simulink model "MultipleAgentsChoice_NoVR"  (Simulink 7.5)
settings: Solver=ode45  StartTime=0.0  StopTime=1000  RelTol=1e-4  AbsTol=1e-4
libraries: simulink x64
(part 1 of 6)
Description:
  | % Copyright (C) 2012 Nicholas K. Lincoln, Sandor M. Veres, Louise Dennis,
  | % Michael Fisher, and Alexei Lisitsa.
  | %
  | % This file is part of the EASS (Engineering Autonomous Space Software)
  | % Demonstrator Set.
  | %
  | % The EASS Demonstrator Set is free software: you can redistribute it
  | % and/or modify it under the terms of the GNU Lesser General Public License
  | % as published by the Free Software Foundation, either version 3 of the
  | % License, or (at your option) any later version.
  | %
  | % The EASS Demonstrator Set is distributed in the hope that it will be
  | % useful, but WITHOUT ANY WARRANTY; without even the implied warranty of
  | % MERCHANTABILITY or FITNESS FOR A PARTICULAR PURPOSE.  See the GNU Lesser
  | % General Public License for more details.
  | %
  | % You should have received a copy of the GNU Lesser General Public License
  | % along with the EASS Demonstrator Set.  If not, see
  | % <http://www.gnu.org/licenses/>.
settings Model: Creator=N K Lincoln  LastModifiedBy=lad
settings SolverCC: ZeroCrossControl=DisableAll
settings OptimizationCC: InitFltsAndDblsToZero=on
settings DebuggingCC: ReadBeforeWriteMsg=DisableAll  WriteAfterWriteMsg=DisableAll  WriteAfterReadMsg=DisableAll  SaveWithParameterizedLinksMsg=none  SignalResolutionControl=TryResolveAllWithWarning  SolverPrmCheckMsg=none  InheritedTsInSrcMsg=none  StrictBusMsg=Warning
settings HardwareCC: TargetHWDeviceType=32-bit Generic
settings GRTTargetCC: TargetFcnLib=ansi_tfl_tmw.mat

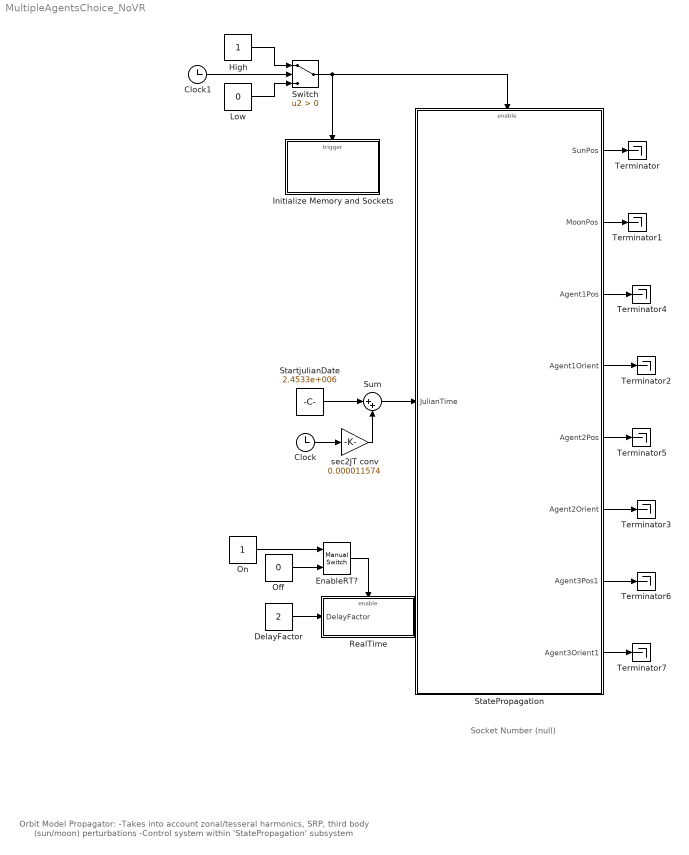
== system MultipleAgentsChoice_NoVR ==
  note: Orbit Model Propagator:
      | -Takes into account zonal/tesseral harmonics, SRP, third body (sun/moon) perturbations
      | -Control system within 'StatePropagation' subsystem
  note: Socket Number (null)
  Clock : Clock
      settings: Decimation=10
  Clock1 : Clock
      settings: Decimation=10
  DelayFactor : Constant  Value=2  OutDataType=sfix(16)  OutScaling=2^0
  EnableRT? : simulink/Signal Routing/Manual Switch  SystemSampleTime=-1  sw=1  action=0  varsize=off
  High : Constant  OutDataType=sfix(16)  OutScaling=2^0
  Initialize Memory and Sockets : Subsystem  TreatAsAtomicUnit=on
  Low : Constant  Value=0  OutDataType=sfix(16)  OutScaling=2^0
  Off : Constant  Value=0  OutDataType=sfix(16)  OutScaling=2^0
  On : Constant  OutDataType=sfix(16)  OutScaling=2^0
  RealTime : Subsystem
  StartjulianDate : Constant  Value=2.4533e+006  OutDataType=sfix(16)  OutScaling=2^0
  StatePropagation : Subsystem
  Sum : Sum  Inputs=|++  OutDataType=sfix(16)  OutScaling=2^0
  Switch : Switch  Criteria=u2 > Threshold
  Terminator{,1..7} (8 alike) : Terminator
  sec2JT conv : Gain  Gain=0.000011574  ParameterDataType=sfix(16)  ParameterScaling=2^0  OutDataType=sfix(16)  OutScaling=2^0
  wires:
  Clock/1 -> sec2JT conv/1
  sec2JT conv/1 -> Sum/2
  Sum/1 -> StatePropagation/1(JulianTime)
  StartjulianDate/1 -> Sum/1
  StatePropagation/7(Agent3Pos1) -> Terminator6/1
  StatePropagation/8(Agent3Orient1) -> Terminator7/1
  StatePropagation/6(Agent2Orient) -> Terminator3/1
  StatePropagation/5(Agent2Pos) -> Terminator5/1
  StatePropagation/4(Agent1Orient) -> Terminator2/1
  StatePropagation/3(Agent1Pos) -> Terminator4/1
  StatePropagation/1(SunPos) -> Terminator/1
  StatePropagation/2(MoonPos) -> Terminator1/1
  On/1 -> EnableRT?/1
  Off/1 -> EnableRT?/2
  EnableRT?/1 -> RealTime/Enable
  DelayFactor/1 -> RealTime/1(DelayFactor)
  Low/1 -> Switch/3
  High/1 -> Switch/1
  Clock1/1 -> Switch/2
  Switch/1 -> StatePropagation/Enable, Initialize Memory and Sockets/Trigger

== system MultipleAgentsChoice_NoVR/Initialize Memory and Sockets ==
  note: number of agents in the cluster
  Trigger : TriggerPort
  Constant : Constant  Value=3  OutDataType=fixdt(1, 16)  OutScaling=2^0
  create multi memory : MATLABFcn  MATLABFcn=create_agent_memory_multi  OutputDimensions=0
  wires:
  Constant/1 -> create multi memory/1

== system MultipleAgentsChoice_NoVR/RealTime ==
  DelayFactor : Inport  OutDataType=sfix(16)  OutScaling=2^0
  Enable : EnablePort
  Real-time synchronization : Subsystem
  wires:
  DelayFactor/1 -> Real-time synchronization/1(DelayFactor)

== system MultipleAgentsChoice_NoVR/StatePropagation ==
  JulianTime : Inport  OutDataType=sfix(16)  OutScaling=2^0
  Enable : EnablePort
  BodyAccelerations : Subsystem
  Bus Selector : BusSelector  OutputSignals=SunPos,MoonPos
  Bus Selector1 : BusSelector  OutputSignals=Agent1Pos,Agent1Vel,Agent2Pos,Agent2Vel,Agent3Pos,Agent3Vel
  MATLAB Fcn : MATLABFcn  MATLABFcn=SatOrient  OutputDimensions=4
  MATLAB Fcn2 : MATLABFcn  MATLABFcn=SatOrient  OutputDimensions=4
  MATLAB Fcn3 : MATLABFcn  MATLABFcn=SatOrient  OutputDimensions=4
  Mux : Mux  Inputs=2
  Mux2 : Mux  Inputs=2
  Mux3 : Mux  Inputs=2
  PropogateAgents : Subsystem
  SatelliteControlAccel : Subsystem
  SunPos : Outport  OutDataType=sfix(16)  OutScaling=2^0
  MoonPos : Outport  Port=2  OutDataType=sfix(16)  OutScaling=2^0
  Agent1Pos : Outport  Port=3  OutDataType=sfix(16)  OutScaling=2^0
  Agent1Orient : Outport  Port=4  OutDataType=sfix(16)  OutScaling=2^0
  Agent2Pos : Outport  Port=5  OutDataType=sfix(16)  OutScaling=2^0
  Agent2Orient : Outport  Port=6  OutDataType=sfix(16)  OutScaling=2^0
  Agent3Pos1 : Outport  Port=7  OutDataType=sfix(16)  OutScaling=2^0
  Agent3Orient1 : Outport  Port=8  OutDataType=sfix(16)  OutScaling=2^0
  wires:
  SatelliteControlAccel/1(AccelControl) -> PropogateAgents/2(ControlAccelrations)
  JulianTime/1 -> BodyAccelerations/1(JulianTime)
  BodyAccelerations/2(SunMoonPos) -> [SunMoonPos]
  BodyAccelerations/1(BodyAccelerations) -> PropogateAgents/1(BodyAccelerations)
  [SunMoonPos] -> Bus Selector/1
  Bus Selector/1 -> SunPos/1  "<SunPos>"
  Bus Selector/2 -> MoonPos/1  "<MoonPos>"
  PropogateAgents/1(GEOC_current) -> Bus Selector1/1, BodyAccelerations/2(GEOC_Current), SatelliteControlAccel/1(GEOC_Current)
  Bus Selector1/1 -> Agent1Pos/1, Mux/1  "<Agent1Pos>"
  Bus Selector1/3 -> Agent2Pos/1, Mux2/1  "<Agent2Pos>"
  Bus Selector1/2 -> Mux/2  "<Agent1Vel>"
  Bus Selector1/4 -> Mux2/2  "<Agent2Vel>"
  Mux/1 -> MATLAB Fcn/1
  Mux2/1 -> MATLAB Fcn2/1
  MATLAB Fcn/1 -> Agent1Orient/1
  MATLAB Fcn2/1 -> Agent2Orient/1
  Bus Selector1/5 -> Mux3/1, Agent3Pos1/1  "<Agent3Pos>"
  Bus Selector1/6 -> Mux3/2  "<Agent3Vel>"
  Mux3/1 -> MATLAB Fcn3/1
  MATLAB Fcn3/1 -> Agent3Orient1/1
  SatelliteControlAccel/2(InitialConditions) -> PropogateAgents/3(InitialConditions)

== system MultipleAgentsChoice_NoVR/RealTime/Real-time synchronization ==
  DelayFactor : Inport  OutDataType=sfix(16)  OutScaling=2^0
  Clock : Clock
      settings: Decimation=10
  Real-time Synchronization : Subsystem
  wires:
  Clock/1 -> Real-time Synchronization/1(run)
  DelayFactor/1 -> Real-time Synchronization/2(DelayFactor)

== system MultipleAgentsChoice_NoVR/StatePropagation/BodyAccelerations ==
  note: THIS IS THE DYNAMIC REGIME INFLUENCING AGENT MOTION
  JulianTime : Inport  OutDataType=sfix(16)  OutScaling=2^0
  GEOC_Current : Inport  Port=2  OutDataType=sfix(16)  OutScaling=2^0
  Agent1 : Subsystem
  Agent2 : Subsystem
  Agent3 : Subsystem
  Bus Creator : BusCreator  Inputs=3
  Bus Creator1 : BusCreator  Inputs=2
  Bus Selector : BusSelector  OutputSignals=Agent1Pos,Agent2Pos,Agent3Pos
  MoonPos : Subsystem
  SunPos : Subsystem
  BodyAccelerations : Outport  OutDataType=sfix(16)  OutScaling=2^0
  SunMoonPos : Outport  Port=2  OutDataType=sfix(16)  OutScaling=2^0
  wires:
  JulianTime/1 -> MoonPos/1(JT), SunPos/1(JT), Agent1/1(JT), Agent2/1(JT), Agent3/1(JT)
  Agent1/1(A1Accels) -> Bus Creator/1  "Agent1"
  Agent2/1(A2Accels) -> Bus Creator/2  "Agent2"
  Bus Creator/1 -> BodyAccelerations/1
  MoonPos/1(MoonGEOC_Pos) -> Bus Creator1/1  "MoonPos"
  SunPos/1(SunPos) -> Bus Creator1/2  "SunPos"
  Bus Creator1/1 -> SunMoonPos/1
  GEOC_Current/1 -> Bus Selector/1
  Bus Selector/1 -> Agent1/2(A1GEOC_Pos)  "<Agent1Pos>"
  Bus Selector/2 -> Agent2/2(A2GEOC_Pos)  "<Agent2Pos>"
  Agent3/1(A3Accels) -> Bus Creator/3  "Agent3"
  Bus Selector/3 -> Agent3/2(A3GEOC_Pos)  "<Agent3Pos>"

== system MultipleAgentsChoice_NoVR/StatePropagation/PropogateAgents ==
  BodyAccelerations : Inport  OutDataType=sfix(16)  OutScaling=2^0
  ControlAccelrations : Inport  Port=2  OutDataType=sfix(16)  OutScaling=2^0
  InitialConditions : Inport  Port=3  OutDataType=sfix(16)  OutScaling=2^0
  Agent1 : Subsystem
  Agent2 : Subsystem
  Agent3 : Subsystem
  Bus Creator : BusCreator  Inputs=6
  Bus Selector : BusSelector  OutputSignals=Agent1,Agent2,Agent3
  Bus Selector1 : BusSelector  OutputSignals=Agent1,Agent2,Agent3
  Bus Selector2 : BusSelector  OutputSignals=ECI_A1,ECI_A2,ECI_A3
  Sum : Sum  Inputs=|++  OutDataType=sfix(16)  OutScaling=2^0
  Sum1 : Sum  Inputs=|++  OutDataType=sfix(16)  OutScaling=2^0
  Sum2 : Sum  Inputs=|++  OutDataType=sfix(16)  OutScaling=2^0
  GEOC_current : Outport  OutDataType=sfix(16)  OutScaling=2^0
  wires:
  BodyAccelerations/1 -> Bus Selector/1
  InitialConditions/1 -> Bus Selector1/1
  Bus Creator/1 -> GEOC_current/1  "GEOC_Current"
  Agent1/1(GEOC_Pos) -> Bus Creator/1  "Agent1Pos"
  Agent2/1(GEOC_Pos) -> Bus Creator/3  "Agent2Pos"
  Agent1/2(GEOC_Vel) -> Bus Creator/2  "Agent1Vel"
  Agent2/2(GEOC_Vel) -> Bus Creator/4  "Agent2Vel"
  ControlAccelrations/1 -> Bus Selector2/1
  Sum/1 -> Agent1/1(Accelerations)
  Sum1/1 -> Agent2/1(Accelerations)
  Bus Selector/1 -> Sum/1  "<Agent1>"
  Bus Selector/2 -> Sum1/1  "<Agent2>"
  Bus Selector2/1 -> Sum/2  "<ECI_A1>"
  Bus Selector2/2 -> Sum1/2  "<ECI_A2>"
  Bus Selector1/2 -> Agent2/2(InitialConditions)  "<Agent2>"
  Bus Selector1/1 -> Agent1/2(InitialConditions)  "<Agent1>"
  Agent3/1(GEOC_Pos) -> Bus Creator/5  "Agent3Pos"
  Agent3/2(GEOC_Vel) -> Bus Creator/6  "Agent3Vel"
  Sum2/1 -> Agent3/1(Accelerations)
  Bus Selector2/3 -> Sum2/2  "<ECI_A3>"
  Bus Selector/3 -> Sum2/1  "<Agent3>"
  Bus Selector1/3 -> Agent3/2(InitialConditions)  "<Agent3>"

== system MultipleAgentsChoice_NoVR/StatePropagation/SatelliteControlAccel ==
  GEOC_Current : Inport  OutDataType=sfix(16)  OutScaling=2^0
  Agent Body1 : Subsystem
  Agent Body2 : Subsystem
  Agent Body3 : Subsystem
  Agent1 : Constant  OutDataType=sfix(16)  OutScaling=2^0
  Agent2 : Constant  Value=2  OutDataType=sfix(16)  OutScaling=2^0
  Agent3 : Constant  Value=3  OutDataType=sfix(16)  OutScaling=2^0
  BodyToOrbitFrameConvert : Subsystem
  Bus Creator : BusCreator  Inputs=3
  Bus Creator1 : BusCreator  Inputs=3
  Bus Selector : BusSelector  OutputSignals=A1Commands,A2Commands,A3Commands,LeadAgent
  Data Type Conversion : DataTypeConversion  OutDataType=sfix(16)  OutScaling=2^0
  Data Type Conversion1 : DataTypeConversion  OutDataType=sfix(16)  OutScaling=2^0
  GetCmdAIL : Subsystem
  InitialErrors : Subsystem
  NoSend : Constant  Value=0  OutDataType=sfix(16)  OutScaling=2^0
  NoSend1 : Constant  Value=0  OutDataType=sfix(16)  OutScaling=2^0
  Pulse Generator : DiscretePulseGenerator  PulseType=Time based  Amplitude=1  Period=1  PulseWidth=50  PhaseDelay=0  SampleTime=1
  Pulse Generator1 : DiscretePulseGenerator  PulseType=Time based  Amplitude=1  Period=0.1  PulseWidth=50  PhaseDelay=0  SampleTime=1
  Selective Hill State Provision and Discretisation : Subsystem
  TriggeredSendAgent : Subsystem  TreatAsAtomicUnit=on
  TriggeredSendCont : Subsystem  TreatAsAtomicUnit=on
  TurnOff : simulink/Signal Routing/Manual Switch  SystemSampleTime=-1  sw=1  action=0  varsize=off
  TurnOff1 : simulink/Signal Routing/Manual Switch  SystemSampleTime=-1  sw=1  action=0  varsize=off
  AccelControl : Outport  OutDataType=sfix(16)  OutScaling=2^0
  InitialConditions : Outport  Port=2  OutDataType=sfix(16)  OutScaling=2^0
  wires:
  BodyToOrbitFrameConvert/1(GlobalAccel) -> AccelControl/1
  GEOC_Current/1 -> Selective Hill State Provision and Discretisation/1(GEOC_Current), BodyToOrbitFrameConvert/3(GEOC_Current)
  Selective Hill State Provision and Discretisation/1(HillState) -> Agent Body1/2(StateInformation), Agent Body2/2(StateInformation), Agent Body3/2(StateInformation)
  Agent Body1/1(AccelA1) -> Bus Creator/1
  Bus Creator/1 -> BodyToOrbitFrameConvert/1(BodyAccel)
  Bus Selector/1 -> Agent Body1/1(Commands)  "<A1Commands>"
  Bus Selector/2 -> Agent Body2/1(Commands)  "<A2Commands>"
  Agent Body2/1(AccelA2) -> Bus Creator/2
  Agent Body1/2(A1Data) -> Bus Creator1/1
  Agent Body2/2(A2Data) -> Bus Creator1/2
  Bus Creator1/1 -> TriggeredSendAgent/1(Data), TriggeredSendCont/1(Data)
  Data Type Conversion/1 -> TriggeredSendAgent/Trigger
  NoSend/1 -> TurnOff/2
  TurnOff/1 -> Data Type Conversion/1
  Pulse Generator/1 -> TurnOff/1
  GetCmdAIL/1(Commands2) -> Bus Selector/1
  Bus Selector/3 -> Agent Body3/1(Commands)  "<A3Commands>"
  Agent Body3/1(AccelA3) -> Bus Creator/3
  Agent Body3/2(A3Data) -> Bus Creator1/3
  Bus Selector/4 -> Selective Hill State Provision and Discretisation/2(LeadAgent), BodyToOrbitFrameConvert/2(LeadAgent)  "<LeadAgent>"
  InitialErrors/1(Out1) -> InitialConditions/1
  Agent2/1 -> Agent Body2/3(AgentNumber)
  Agent3/1 -> Agent Body3/3(AgentNumber)
  Agent1/1 -> Agent Body1/3(AgentNumber)
  NoSend1/1 -> TurnOff1/2
  TurnOff1/1 -> Data Type Conversion1/1
  Pulse Generator1/1 -> TurnOff1/1
  Data Type Conversion1/1 -> TriggeredSendCont/Trigger

== system MultipleAgentsChoice_NoVR/RealTime/Real-time synchronization/Real-time Synchronization ==
  run : Inport
  DelayFactor : Inport  Port=2  OutDataType=sfix(16)  OutScaling=2^0
  Clock : Clock
      settings: Decimation=10
  Product : Product  OutDataType=sfix(16)  OutScaling=2^0  RndMeth=Zero
  Subsystem : Subsystem  TreatAsAtomicUnit=on
  Sum : Sum  Inputs=+-  SaturateOnIntegerOverflow=on  InputSameDT=on  OutDataTypeStr=Inherit: Same as first input
  real-time synchronization : MATLABFcn  MATLABFcn=waitfortreal  OutputDimensions=0
  wires:
  run/1 -> Subsystem/Trigger
  Subsystem/1(Out) -> Sum/2
  Clock/1 -> Sum/1, Subsystem/1(In)
  Sum/1 -> Product/2
  Product/1 -> real-time synchronization/1
  DelayFactor/1 -> Product/1

== system MultipleAgentsChoice_NoVR/StatePropagation/BodyAccelerations/Agent1 ==
  JT : Inport  OutDataType=sfix(16)  OutScaling=2^0
  A1GEOC_Pos : Inport  Port=2  OutDataType=sfix(16)  OutScaling=2^0
  EarthAccel(J2) : Subsystem
  EarthAccel1 : Subsystem
  Gain{,1..3,5} (5 alike) : Gain  ParameterDataType=sfix(16)  ParameterScaling=2^0  OutDataType=sfix(16)  OutScaling=2^0
  Manual Switch : simulink/Signal Routing/Manual Switch  SystemSampleTime=-1  sw=1  action=0  varsize=off
  MoonAccel : Subsystem
  SRPAccel : Subsystem
  Sum : Sum  Inputs=|++++  OutDataType=sfix(16)  OutScaling=2^0
  SunAccel : Subsystem
  A1Accels : Outport  OutDataType=sfix(16)  OutScaling=2^0
  wires:
  EarthAccel(J2)/1(AccelEarth) -> Gain/1
  MoonAccel/1(AccelMoon) -> Gain1/1
  SRPAccel/1(AccelSRP) -> Gain2/1
  SunAccel/1(AccelSun) -> Gain5/1
  EarthAccel1/1(AccelEarth) -> Gain3/1
  A1GEOC_Pos/1 -> EarthAccel1/1(GEOC_Pos), EarthAccel(J2)/2(GEOC_Pos), MoonAccel/2(SatGEOC_Pos), SRPAccel/2(GEOC_Pos1), SunAccel/2(SatGEOC_Pos1)
  JT/1 -> EarthAccel(J2)/1(JT), MoonAccel/1(JT), SRPAccel/1(JT1), SunAccel/1(JT1)
  Gain/1 -> Sum/1
  Gain1/1 -> Sum/2
  Gain2/1 -> Sum/3
  Gain5/1 -> Sum/4
  Sum/1 -> Manual Switch/2
  Manual Switch/1 -> A1Accels/1
  Gain3/1 -> Manual Switch/1

== system MultipleAgentsChoice_NoVR/StatePropagation/BodyAccelerations/Agent2 ==
  JT : Inport  OutDataType=sfix(16)  OutScaling=2^0
  A2GEOC_Pos : Inport  Port=2  OutDataType=sfix(16)  OutScaling=2^0
  EarthAccel(J2) : Subsystem
  EarthAccel1 : Subsystem
  Gain{,1..3,5} (5 alike) : Gain  ParameterDataType=sfix(16)  ParameterScaling=2^0  OutDataType=sfix(16)  OutScaling=2^0
  Manual Switch : simulink/Signal Routing/Manual Switch  SystemSampleTime=-1  sw=1  action=0  varsize=off
  MoonAccel : Subsystem
  SRPAccel : Subsystem
  Sum : Sum  Inputs=|++++  OutDataType=sfix(16)  OutScaling=2^0
  SunAccel : Subsystem
  A2Accels : Outport  OutDataType=sfix(16)  OutScaling=2^0
  wires:
  Gain3/1 -> Manual Switch/1
  Manual Switch/1 -> A2Accels/1
  Sum/1 -> Manual Switch/2
  Gain5/1 -> Sum/4
  Gain2/1 -> Sum/3
  Gain1/1 -> Sum/2
  Gain/1 -> Sum/1
  JT/1 -> SunAccel/1(JT1), SRPAccel/1(JT1), MoonAccel/1(JT), EarthAccel(J2)/1(JT)
  A2GEOC_Pos/1 -> SunAccel/2(SatGEOC_Pos1), SRPAccel/2(GEOC_Pos1), MoonAccel/2(SatGEOC_Pos), EarthAccel(J2)/2(GEOC_Pos), EarthAccel1/1(GEOC_Pos)
  EarthAccel1/1(AccelEarth) -> Gain3/1
  SunAccel/1(AccelSun) -> Gain5/1
  SRPAccel/1(AccelSRP) -> Gain2/1
  MoonAccel/1(AccelMoon) -> Gain1/1
  EarthAccel(J2)/1(AccelEarth) -> Gain/1

== system MultipleAgentsChoice_NoVR/StatePropagation/BodyAccelerations/Agent3 ==
  JT : Inport  OutDataType=sfix(16)  OutScaling=2^0
  A3GEOC_Pos : Inport  Port=2  OutDataType=sfix(16)  OutScaling=2^0
  EarthAccel(J2) : Subsystem
  EarthAccel1 : Subsystem
  Gain{,1..3,5} (5 alike) : Gain  ParameterDataType=sfix(16)  ParameterScaling=2^0  OutDataType=sfix(16)  OutScaling=2^0
  Manual Switch : simulink/Signal Routing/Manual Switch  SystemSampleTime=-1  sw=1  action=0  varsize=off
  MoonAccel : Subsystem
  SRPAccel : Subsystem
  Sum : Sum  Inputs=|++++  OutDataType=sfix(16)  OutScaling=2^0
  SunAccel : Subsystem
  A3Accels : Outport  OutDataType=sfix(16)  OutScaling=2^0
  wires:
  EarthAccel(J2)/1(AccelEarth) -> Gain/1
  MoonAccel/1(AccelMoon) -> Gain1/1
  SRPAccel/1(AccelSRP) -> Gain2/1
  SunAccel/1(AccelSun) -> Gain5/1
  EarthAccel1/1(AccelEarth) -> Gain3/1
  A3GEOC_Pos/1 -> EarthAccel1/1(GEOC_Pos), EarthAccel(J2)/2(GEOC_Pos), MoonAccel/2(SatGEOC_Pos), SRPAccel/2(GEOC_Pos1), SunAccel/2(SatGEOC_Pos1)
  JT/1 -> EarthAccel(J2)/1(JT), MoonAccel/1(JT), SRPAccel/1(JT1), SunAccel/1(JT1)
  Gain/1 -> Sum/1
  Gain1/1 -> Sum/2
  Gain2/1 -> Sum/3
  Gain5/1 -> Sum/4
  Sum/1 -> Manual Switch/2
  Manual Switch/1 -> A3Accels/1
  Gain3/1 -> Manual Switch/1

== system MultipleAgentsChoice_NoVR/StatePropagation/BodyAccelerations/MoonPos ==
  JT : Inport  OutDataType=sfix(16)  OutScaling=2^0
  MoonDirVector : MATLABFcn  MATLABFcn=moon
  Re : Gain  Gain=6371  ParameterDataType=sfix(16)  ParameterScaling=2^0  OutDataType=sfix(16)  OutScaling=2^0
  MoonGEOC_Pos : Outport  OutDataType=sfix(16)  OutScaling=2^0
  wires:
  Re/1 -> MoonGEOC_Pos/1
  MoonDirVector/1 -> Re/1
  JT/1 -> MoonDirVector/1

== system MultipleAgentsChoice_NoVR/StatePropagation/BodyAccelerations/SunPos ==
  JT : Inport  OutDataType=sfix(16)  OutScaling=2^0
  AU : Gain  Gain=1.4960e8  ParameterDataType=sfix(16)  ParameterScaling=2^0  OutDataType=sfix(16)  OutScaling=2^0
  SunDirVector : MATLABFcn  MATLABFcn=sun
  SunPos : Outport  OutDataType=sfix(16)  OutScaling=2^0
  wires:
  AU/1 -> SunPos/1
  SunDirVector/1 -> AU/1
  JT/1 -> SunDirVector/1

== system MultipleAgentsChoice_NoVR/StatePropagation/PropogateAgents/Agent1 ==
  Accelerations : Inport  OutDataType=sfix(16)  OutScaling=2^0
  InitialConditions : Inport  Port=2  OutDataType=sfix(16)  OutScaling=2^0
  Demux : Demux  Outputs=6
  Integrate2Pos : Integrator  InitialConditionSource=external
  Integrate2Vel : Integrator  InitialConditionSource=external
  Mux : Mux  Inputs=3
  Mux1 : Mux  Inputs=3
  GEOC_Pos : Outport  OutDataType=sfix(16)  OutScaling=2^0
  GEOC_Vel : Outport  Port=2  OutDataType=sfix(16)  OutScaling=2^0
  wires:
  Integrate2Vel/1 -> Integrate2Pos/1, GEOC_Vel/1
  Accelerations/1 -> Integrate2Vel/1
  Demux/1 -> Mux/1
  Demux/2 -> Mux/2
  Demux/3 -> Mux/3
  Demux/4 -> Mux1/1
  Demux/5 -> Mux1/2
  Demux/6 -> Mux1/3
  InitialConditions/1 -> Demux/1
  Mux1/1 -> Integrate2Vel/2
  Mux/1 -> Integrate2Pos/2
  Integrate2Pos/1 -> GEOC_Pos/1

== system MultipleAgentsChoice_NoVR/StatePropagation/PropogateAgents/Agent2 ==
  Accelerations : Inport  OutDataType=sfix(16)  OutScaling=2^0
  InitialConditions : Inport  Port=2  OutDataType=sfix(16)  OutScaling=2^0
  Demux : Demux  Outputs=6
  Integrate2Pos : Integrator  InitialConditionSource=external
  Integrate2Vel : Integrator  InitialConditionSource=external
  Mux : Mux  Inputs=3
  Mux1 : Mux  Inputs=3
  GEOC_Pos : Outport  OutDataType=sfix(16)  OutScaling=2^0
  GEOC_Vel : Outport  Port=2  OutDataType=sfix(16)  OutScaling=2^0
  wires:
  Integrate2Pos/1 -> GEOC_Pos/1
  Mux/1 -> Integrate2Pos/2
  Mux1/1 -> Integrate2Vel/2
  InitialConditions/1 -> Demux/1
  Demux/6 -> Mux1/3
  Demux/5 -> Mux1/2
  Demux/4 -> Mux1/1
  Demux/3 -> Mux/3
  Demux/2 -> Mux/2
  Demux/1 -> Mux/1
  Accelerations/1 -> Integrate2Vel/1
  Integrate2Vel/1 -> GEOC_Vel/1, Integrate2Pos/1

== system MultipleAgentsChoice_NoVR/StatePropagation/PropogateAgents/Agent3 ==
  Accelerations : Inport  OutDataType=sfix(16)  OutScaling=2^0
  InitialConditions : Inport  Port=2  OutDataType=sfix(16)  OutScaling=2^0
  Demux : Demux  Outputs=6
  Integrate2Pos : Integrator  InitialConditionSource=external
  Integrate2Vel : Integrator  InitialConditionSource=external
  Mux : Mux  Inputs=3
  Mux1 : Mux  Inputs=3
  GEOC_Pos : Outport  OutDataType=sfix(16)  OutScaling=2^0
  GEOC_Vel : Outport  Port=2  OutDataType=sfix(16)  OutScaling=2^0
  wires:
  Integrate2Vel/1 -> Integrate2Pos/1, GEOC_Vel/1
  Accelerations/1 -> Integrate2Vel/1
  Demux/1 -> Mux/1
  Demux/2 -> Mux/2
  Demux/3 -> Mux/3
  Demux/4 -> Mux1/1
  Demux/5 -> Mux1/2
  Demux/6 -> Mux1/3
  InitialConditions/1 -> Demux/1
  Mux1/1 -> Integrate2Vel/2
  Mux/1 -> Integrate2Pos/2
  Integrate2Pos/1 -> GEOC_Pos/1

== system MultipleAgentsChoice_NoVR/StatePropagation/SatelliteControlAccel/Agent Body1 ==
  note: 1=sequence running
  note: 0=no sequence ruinning
  Commands : Inport  OutDataType=sfix(16)  OutScaling=2^0
  StateInformation : Inport  Port=2  OutDataType=sfix(16)  OutScaling=2^0
  AgentNumber : Inport  Port=3  OutDataType=sfix(16)  OutScaling=2^0
  Actual Thruster response : Subsystem
  ActualForces : Display
  AgentNumber1 : InportShadow  Port=3  OutDataType=sfix(16)  OutScaling=2^0
  Bus Creator : BusCreator  Inputs=9
  Bus Creator1 : BusCreator  Inputs=2
  Bus Creator2 : BusCreator  Inputs=9
  Bus Selector : BusSelector  OutputSignals=ControlType,UseX,UseY,UseZ,UseXYZ,XValves1,XSwitch1,YValves,YSwitch,ZValves,ZSwitch,XYZValves,XYZSwitch,A1Break
  Bus Selector1 : BusSelector  OutputSignals=A1HillState.HillPosCont,A1HillState.HillVelCont,A1HillState.HillPosDisc,A1HillState.HillVelDisc
  Clock : Clock
      settings: Decimation=10
  Constant : Constant  Value=[0;0;0]  OutDataType=sfix(16)  OutScaling=2^0
  Convert2Accels : Subsystem
  Demux : Demux  Outputs=8
  Derivative : Derivative
  DesiredForces : Display
  Mux : Mux  Inputs=6
  Mux1 : Mux
  Mux2 : Mux
  Mux3 : Mux  Inputs=3
  Mux4 : Mux  Inputs=2
  Mux5 : Mux  Inputs=2
  Plan : Display
  Sum : Sum  Inputs=|++  OutDataType=sfix(16)  OutScaling=2^0
  obtain_forcesXYZ_multi : MATLABFcn  MATLABFcn=obtain_forcesXYZ_multi  OutputDimensions=8
  AccelA1 : Outport  OutDataType=sfix(16)  OutScaling=2^0
  A1Data : Outport  Port=2  OutDataType=sfix(16)  OutScaling=2^0
  wires:
  Derivative/1 -> Mux/3
  Clock/1 -> Mux/4
  [CTstate] -> Derivative/1, Mux/2
  obtain_forcesXYZ_multi/1 -> Demux/1
  Mux/1 -> obtain_forcesXYZ_multi/1
  Bus Creator1/1 -> Actual Thruster response/1(Signals)
  Commands/1 -> Bus Selector/1
  Actual Thruster response/5(Forces) -> Bus Creator2/7, Sum/1, ActualForces/1  "A1ActualForces"
  Mux1/1 -> Bus Creator1/1  "A1ControlSignals"
  StateInformation/1 -> Bus Selector1/1
  Bus Selector1/1 -> Mux4/1  "<HillPosCont>"
  Bus Selector1/2 -> Mux4/2  "<HillVelCont>"
  Bus Selector1/3 -> Mux5/1  "<HillPosDisc>"
  Bus Selector1/4 -> Mux5/2  "<HillVelDisc>"
  Mux5/1 -> [DTstate]
  Mux4/1 -> [CTstate]
  Convert2Accels/1(Accels) -> AccelA1/1  "A1Accels"
  Actual Thruster response/2(YThrusterData) -> Bus Creator2/4  "A1YthrusterData"
  Actual Thruster response/1(XThrusterData) -> Bus Creator2/3  "A1XthrusterData"
  Actual Thruster response/3(ZThrusterData) -> Bus Creator2/5  "A1ZthrusterData"
  Demux/1 -> Bus Creator2/1, Plan/1  "A1PlanMsg"
  Bus Creator2/1 -> A1Data/1  "A1Data"
  [DTstate] -> Bus Creator2/9  "A1DTstate"
  Actual Thruster response/4(XYZThrusterData) -> Bus Creator2/6  "A1XYZthrusterData"
  Bus Selector/1 -> Mux/1  "<ControlType>"
  Bus Selector/2 -> Mux2/1  "<UseX>"
  Bus Selector/3 -> Mux2/2  "<UseY>"
  Bus Selector/4 -> Mux2/3  "<UseZ>"
  Bus Selector/5 -> Mux2/4  "<UseXYZ>"
  Mux2/1 -> Mux/5
  Bus Creator/1 -> Bus Creator1/2  "ConfigurationSignals"
  Bus Selector/6 -> Bus Creator/1  "<XValves1>"
  Bus Selector/7 -> Bus Creator/2  "<XSwitch1>"
  Bus Selector/8 -> Bus Creator/3  "<YValves>"
  Bus Selector/9 -> Bus Creator/4  "<YSwitch>"
  Bus Selector/10 -> Bus Creator/5  "<ZValves>"
  Bus Selector/11 -> Bus Creator/6  "<ZSwitch>"
  Bus Selector/12 -> Bus Creator/7  "<XYZValves>"
  Bus Selector/13 -> Bus Creator/8  "<XYZSwitch>"
  Demux/2 -> Mux3/1
  Demux/3 -> Mux3/2
  Demux/4 -> Mux3/3
  Demux/5 -> Mux1/1
  Demux/6 -> Mux1/2
  Demux/7 -> Mux1/3
  Demux/8 -> Mux1/4
  Mux3/1 -> Bus Creator2/2, DesiredForces/1  "A1DesiredForces"
  Sum/1 -> Convert2Accels/1(Forces)
  Constant/1 -> Sum/2
  AgentNumber/1 -> Mux/6
  AgentNumber1/1 -> Actual Thruster response/2(AgentNumber)
  Actual Thruster response/6(PressureData) -> Bus Creator2/8  "A1PressureData"
  Bus Selector/14 -> Bus Creator/9  "<A1Break>"

== system MultipleAgentsChoice_NoVR/StatePropagation/SatelliteControlAccel/Agent Body2 ==
  Commands : Inport  OutDataType=sfix(16)  OutScaling=2^0
  StateInformation : Inport  Port=2  OutDataType=sfix(16)  OutScaling=2^0
  AgentNumber : Inport  Port=3  OutDataType=sfix(16)  OutScaling=2^0
  Actual Thruster response : Subsystem
  AgentNumber1 : InportShadow  Port=3  OutDataType=sfix(16)  OutScaling=2^0
  Bus Creator : BusCreator  Inputs=9
  Bus Creator1 : BusCreator  Inputs=2
  Bus Creator2 : BusCreator  Inputs=9
  Bus Selector : BusSelector  OutputSignals=ControlType,UseX,UseY,UseZ,UseXYZ,XValves1,XSwitch1,YValves,YSwitch,ZValves,ZSwitch,XYZValves,XYZSwitch,A2Break
  Bus Selector1 : BusSelector  OutputSignals=A2HillState.HillPosCont,A2HillState.HillVelCont,A2HillState.HillPosDisc,A2HillState.HillVelDisc
  Clock : Clock
      settings: Decimation=10
  Convert2Accels : Subsystem
  Demux : Demux  Outputs=8
  Derivative : Derivative
  Mux : Mux  Inputs=6
  Mux1 : Mux
  Mux2 : Mux
  Mux3 : Mux  Inputs=3
  Mux4 : Mux  Inputs=2
  Mux5 : Mux  Inputs=2
  obtain_forcesXYZ_multi : MATLABFcn  MATLABFcn=obtain_forcesXYZ_multi  OutputDimensions=8
  AccelA2 : Outport  OutDataType=sfix(16)  OutScaling=2^0
  A2Data : Outport  Port=2  OutDataType=sfix(16)  OutScaling=2^0
  wires:
  Bus Selector/13 -> Bus Creator/8  "<XYZSwitch>"
  Bus Selector/12 -> Bus Creator/7  "<XYZValves>"
  Bus Selector/11 -> Bus Creator/6  "<ZSwitch>"
  Bus Selector/10 -> Bus Creator/5  "<ZValves>"
  Bus Selector/9 -> Bus Creator/4  "<YSwitch>"
  Bus Selector/8 -> Bus Creator/3  "<YValves>"
  Bus Selector/7 -> Bus Creator/2  "<XSwitch1>"
  Bus Selector/6 -> Bus Creator/1  "<XValves1>"
  Bus Creator/1 -> Bus Creator1/2  "ConfigurationSignals"
  Mux2/1 -> Mux/5
  Bus Selector/5 -> Mux2/4  "<UseXYZ>"
  Bus Selector/4 -> Mux2/3  "<UseZ>"
  Bus Selector/3 -> Mux2/2  "<UseY>"
  Bus Selector/2 -> Mux2/1  "<UseX>"
  Bus Selector/1 -> Mux/1  "<ControlType>"
  Actual Thruster response/4(XYZThrusterData) -> Bus Creator2/6  "A2XYZthrusterData"
  [DTstate] -> Bus Creator2/9  "A2DTstate"
  Bus Creator2/1 -> A2Data/1  "A2Data"
  Actual Thruster response/3(ZThrusterData) -> Bus Creator2/5  "A2ZthrusterData"
  Actual Thruster response/1(XThrusterData) -> Bus Creator2/3  "A2XthrusterData"
  Actual Thruster response/2(YThrusterData) -> Bus Creator2/4  "A2YthrusterData"
  Convert2Accels/1(Accels) -> AccelA2/1  "A2Accels"
  Mux4/1 -> [CTstate]
  Mux5/1 -> [DTstate]
  Bus Selector1/4 -> Mux5/2  "<HillVelDisc>"
  Bus Selector1/3 -> Mux5/1  "<HillPosDisc>"
  Bus Selector1/2 -> Mux4/2  "<HillVelCont>"
  Bus Selector1/1 -> Mux4/1  "<HillPosCont>"
  StateInformation/1 -> Bus Selector1/1
  Mux1/1 -> Bus Creator1/1  "A2ControlSignals"
  Actual Thruster response/5(Forces) -> Convert2Accels/1(Forces), Bus Creator2/7  "A2ActualForces"
  Commands/1 -> Bus Selector/1
  Bus Creator1/1 -> Actual Thruster response/1(Signals)
  Mux/1 -> obtain_forcesXYZ_multi/1
  obtain_forcesXYZ_multi/1 -> Demux/1
  [CTstate] -> Derivative/1, Mux/2
  Clock/1 -> Mux/4
  Derivative/1 -> Mux/3
  Demux/1 -> Bus Creator2/1  "A2PlanMsg"
  Demux/2 -> Mux3/1
  Demux/3 -> Mux3/2
  Demux/4 -> Mux3/3
  Demux/5 -> Mux1/1
  Demux/6 -> Mux1/2
  Demux/7 -> Mux1/3
  Demux/8 -> Mux1/4
  Mux3/1 -> Bus Creator2/2  "A2DesiredForces"
  AgentNumber/1 -> Mux/6
  AgentNumber1/1 -> Actual Thruster response/2(AgentNumber)
  Actual Thruster response/6(PressureData) -> Bus Creator2/8  "A2PressureData"
  Bus Selector/14 -> Bus Creator/9  "<A2Break>"

== system MultipleAgentsChoice_NoVR/StatePropagation/SatelliteControlAccel/Agent Body3 ==
  note: 1=sequence running
  note: 0=no sequence ruinning
  Commands : Inport  OutDataType=sfix(16)  OutScaling=2^0
  StateInformation : Inport  Port=2  OutDataType=sfix(16)  OutScaling=2^0
  AgentNumber : Inport  Port=3  OutDataType=sfix(16)  OutScaling=2^0
  Actual Thruster response : Subsystem
  AgentNumber1 : InportShadow  Port=3  OutDataType=sfix(16)  OutScaling=2^0
  Bus Creator : BusCreator  Inputs=9
  Bus Creator1 : BusCreator  Inputs=2
  Bus Creator2 : BusCreator  Inputs=9
  Bus Selector : BusSelector  OutputSignals=ControlType,UseX,UseY,UseZ,UseXYZ,XValves1,XSwitch1,YValves,YSwitch,ZValves,ZSwitch,XYZValves,XYZSwitch,A3Break
  Bus Selector1 : BusSelector  OutputSignals=A3HillState.HillPosCont,A3HillState.HillVelCont,A3HillState.HillPosDisc,A3HillState.HillVelDisc
  Clock : Clock
      settings: Decimation=10
  Convert2Accels : Subsystem
  Demux : Demux  Outputs=8
  Derivative : Derivative
  Mux : Mux  Inputs=6
  Mux1 : Mux
  Mux2 : Mux
  Mux3 : Mux  Inputs=3
  Mux4 : Mux  Inputs=2
  Mux5 : Mux  Inputs=2
  obtain_forcesXYZ_multi : MATLABFcn  MATLABFcn=obtain_forcesXYZ_multi  OutputDimensions=8
  AccelA3 : Outport  OutDataType=sfix(16)  OutScaling=2^0
  A3Data : Outport  Port=2  OutDataType=sfix(16)  OutScaling=2^0
  wires:
  Mux3/1 -> Bus Creator2/2  "A3DesiredForces"
  Demux/8 -> Mux1/4
  Demux/7 -> Mux1/3
  Demux/6 -> Mux1/2
  Demux/5 -> Mux1/1
  Demux/4 -> Mux3/3
  Demux/3 -> Mux3/2
  Demux/2 -> Mux3/1
  Demux/1 -> Bus Creator2/1  "A3PlanMsg"
  Derivative/1 -> Mux/3
  Clock/1 -> Mux/4
  [CTstate] -> Derivative/1, Mux/2
  obtain_forcesXYZ_multi/1 -> Demux/1
  Mux/1 -> obtain_forcesXYZ_multi/1
  Bus Creator1/1 -> Actual Thruster response/1(Signals)
  Commands/1 -> Bus Selector/1
  Actual Thruster response/5(Forces) -> Bus Creator2/7, Convert2Accels/1(Forces)  "A3ActualForces"
  Mux1/1 -> Bus Creator1/1  "A3ControlSignals"
  StateInformation/1 -> Bus Selector1/1
  Bus Selector1/1 -> Mux4/1  "<HillPosCont>"
  Bus Selector1/2 -> Mux4/2  "<HillVelCont>"
  Bus Selector1/3 -> Mux5/1  "<HillPosDisc>"
  Bus Selector1/4 -> Mux5/2  "<HillVelDisc>"
  Mux5/1 -> [DTstate]
  Mux4/1 -> [CTstate]
  Convert2Accels/1(Accels) -> AccelA3/1  "A3Accels"
  Actual Thruster response/2(YThrusterData) -> Bus Creator2/4  "A3YthrusterData"
  Actual Thruster response/1(XThrusterData) -> Bus Creator2/3  "A3XthrusterData"
  Actual Thruster response/3(ZThrusterData) -> Bus Creator2/5  "A3ZthrusterData"
  Bus Creator2/1 -> A3Data/1  "A3Data"
  [DTstate] -> Bus Creator2/9  "A3DTstate"
  Actual Thruster response/4(XYZThrusterData) -> Bus Creator2/6  "A3XYZthrusterData"
  Bus Selector/1 -> Mux/1  "<ControlType>"
  Bus Selector/2 -> Mux2/1  "<UseX>"
  Bus Selector/3 -> Mux2/2  "<UseY>"
  Bus Selector/4 -> Mux2/3  "<UseZ>"
  Bus Selector/5 -> Mux2/4  "<UseXYZ>"
  Mux2/1 -> Mux/5
  Bus Creator/1 -> Bus Creator1/2  "ConfigurationSignals"
  Bus Selector/6 -> Bus Creator/1  "<XValves1>"
  Bus Selector/7 -> Bus Creator/2  "<XSwitch1>"
  Bus Selector/8 -> Bus Creator/3  "<YValves>"
  Bus Selector/9 -> Bus Creator/4  "<YSwitch>"
  Bus Selector/10 -> Bus Creator/5  "<ZValves>"
  Bus Selector/11 -> Bus Creator/6  "<ZSwitch>"
  Bus Selector/12 -> Bus Creator/7  "<XYZValves>"
  Bus Selector/13 -> Bus Creator/8  "<XYZSwitch>"
  AgentNumber/1 -> Mux/6
  AgentNumber1/1 -> Actual Thruster response/2(AgentNumber)
  Actual Thruster response/6(PressureData) -> Bus Creator2/8  "A3PressureData"
  Bus Selector/14 -> Bus Creator/9  "<A3Break>"

== system MultipleAgentsChoice_NoVR/StatePropagation/SatelliteControlAccel/BodyToOrbitFrameConvert ==
  BodyAccel : Inport  OutDataType=sfix(16)  OutScaling=2^0
  LeadAgent : Inport  Port=2  OutDataType=sfix(16)  OutScaling=2^0
  GEOC_Current : Inport  Port=3  OutDataType=sfix(16)  OutScaling=2^0
  Bus Creator : BusCreator  Inputs=3
  Bus Selector : BusSelector  OutputSignals=A1Accels,A2Accels,A3Accels
  Bus Selector2 : BusSelector  OutputSignals=Agent1Pos,Agent1Vel,Agent2Pos,Agent2Vel,Agent3Pos,Agent3Vel
  Hill2ECI_A1 : MATLABFcn  MATLABFcn=Hill2ECI  OutputDimensions=3
  Hill2ECI_A2 : MATLABFcn  MATLABFcn=Hill2ECI  OutputDimensions=3
  Hill2ECI_A3 : MATLABFcn  MATLABFcn=Hill2ECI  OutputDimensions=3
  Multiport Switch : MultiPortSwitch  zeroidx=off
  Mux{,1..2,4..6} (6 alike) : Mux  Inputs=2
  GlobalAccel : Outport  OutDataType=sfix(16)  OutScaling=2^0
  wires:
  BodyAccel/1 -> Bus Selector/1
  Mux/1 -> Hill2ECI_A1/1
  Mux1/1 -> Hill2ECI_A2/1
  Bus Selector/1 -> Mux/1  "<A1Accels>"
  Bus Selector/2 -> Mux1/1  "<A2Accels>"
  Hill2ECI_A1/1 -> Bus Creator/1  "ECI_A1"
  Hill2ECI_A2/1 -> Bus Creator/2  "ECI_A2"
  Bus Creator/1 -> GlobalAccel/1  "ECI_Accels"
  Hill2ECI_A3/1 -> Bus Creator/3  "ECI_A3"
  Mux2/1 -> Hill2ECI_A3/1
  Bus Selector/3 -> Mux2/1  "<A3Accels>"
  Multiport Switch/1 -> Mux1/2, Mux2/2, Mux/2
  Mux6/1 -> Multiport Switch/4
  Mux5/1 -> Multiport Switch/3
  Mux4/1 -> Multiport Switch/2
  Bus Selector2/6 -> Mux6/2  "<Agent3Vel>"
  Bus Selector2/5 -> Mux6/1  "<Agent3Pos>"
  Bus Selector2/4 -> Mux5/2  "<Agent2Vel>"
  Bus Selector2/3 -> Mux5/1  "<Agent2Pos>"
  Bus Selector2/2 -> Mux4/2  "<Agent1Vel>"
  Bus Selector2/1 -> Mux4/1  "<Agent1Pos>"
  GEOC_Current/1 -> Bus Selector2/1
  LeadAgent/1 -> Multiport Switch/1
